simulink model "code"  (R2018b)
settings: Solver=VariableStepAuto  StartTime=0.0  StopTime=40.0  RelTol=1e-3
settings Model: Creator=Shubhi  LastModifiedBy=Shubhi

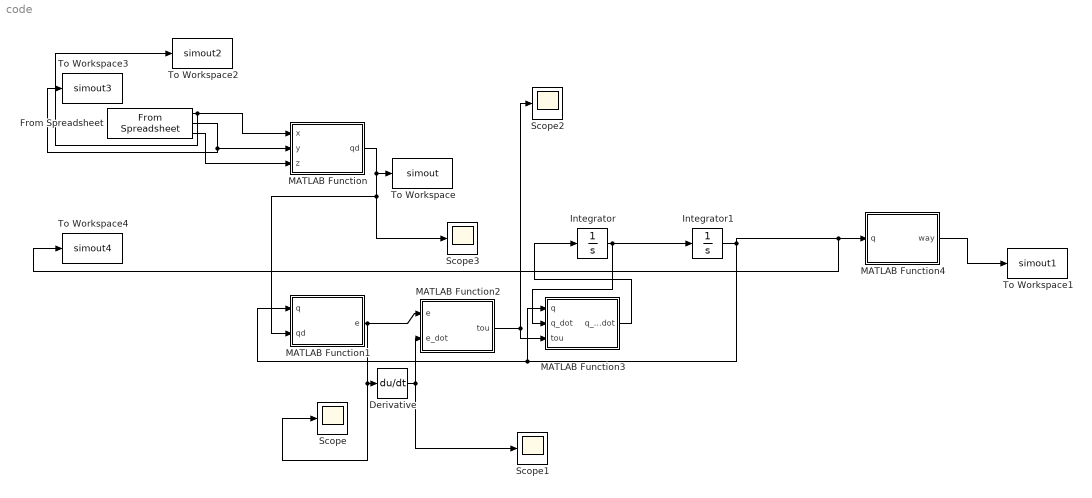
== system code ==
  Derivative : Derivative
  From Spreadsheet : FromSpreadsheet  FileName=C:\Users\Shubhi\Downloads\testdata.xlsx  SampleTime=0.5
  Integrator : Integrator  InitialCondition=[0;0;0;0]
  Integrator1 : Integrator  InitialCondition=[0;0;0;0]
  MATLAB Function : MATLAB Function  TreatAsAtomicUnit=on
  MATLAB Function1 : MATLAB Function  TreatAsAtomicUnit=on
  MATLAB Function2 : MATLAB Function  TreatAsAtomicUnit=on
  MATLAB Function3 : MATLAB Function  TreatAsAtomicUnit=on
  MATLAB Function4 : MATLAB Function  TreatAsAtomicUnit=on
  Scope{,1..3} (4 alike) : Scope
  To Workspace : ToWorkspace  VariableName=simout  SaveFormat=Timeseries  SampleTime=-1
  To Workspace1 : ToWorkspace  VariableName=simout1  SaveFormat=Timeseries  SampleTime=-1
  To Workspace2 : ToWorkspace  VariableName=simout2  SaveFormat=Timeseries  SampleTime=-1
  To Workspace3 : ToWorkspace  VariableName=simout3  SaveFormat=Timeseries  SampleTime=-1
  To Workspace4 : ToWorkspace  VariableName=simout4  SaveFormat=Timeseries  SampleTime=-1
  wires:
  From Spreadsheet/1 -> To Workspace2/1, MATLAB Function/1(x)
  From Spreadsheet/3 -> MATLAB Function/3(z)
  From Spreadsheet/2 -> To Workspace3/1, MATLAB Function/2(y)
  MATLAB Function/1(qd) -> Scope3/1, MATLAB Function1/2(qd), To Workspace/1
  MATLAB Function1/1(e) -> Scope/1, Derivative/1, MATLAB Function2/1(e)
  Derivative/1 -> Scope1/1, MATLAB Function2/2(e_dot)
  MATLAB Function2/1(tou) -> Scope2/1, MATLAB Function3/3(tou)
  Integrator/1 -> MATLAB Function3/2(q_dot), Integrator1/1
  MATLAB Function3/1(q_double_dot) -> Integrator/1
  Integrator1/1 -> To Workspace4/1, MATLAB Function4/1(q), MATLAB Function1/1(q), MATLAB Function3/1(q)
  MATLAB Function4/1(way) -> To Workspace1/1

== matlab function code/MATLAB Function1 ==
  data: q input; e output; qd input
function e=fcn(q, qd)
e=q-qd;

== matlab function code/MATLAB Function ==
  data: x input; qd output; y input; z input
function qd = fcn(x,y,z) 
l1=0.2;
l2=0.25;
theta1=acos(x/(x*x+y*y)^0.5) - acos((x^2+y^2+l1^2-l2^2)/(2*l1*(x^2+y^2)^(1/2))); 
theta2=acos(((x^2+y^2-l1^2-l2^2)/(2*l1*l2)));      
l0=0;

%a=y<0.2 | x<0;
%qd=[((-1)^(1+a)).*theta1;((-1)^(1+a)).*theta2;0;z-l0];
qd=[theta1;theta2;0;z-l0];

== matlab function code/MATLAB Function2 ==
  data: e input; tou output; e_dot input
function tou = fcn(e,e_dot)

 tou = -20*e-20*e_dot;

== matlab function code/MATLAB Function3 ==
  data: q_double_dot output; q input; q_dot input; tou input
function q_double_dot = fcn(q,q_dot,tou)

m1 = 20;
m2 = 15;
m3 = 15;
m4 = 0.5; 
 
l1 = 0.2;
l2 = 0.25; 
r1 = 0.1;
r2 = 0.125;

Iz1 = 0.27 ; 
 Iz2= 0.31;
Iz3 = 0.02;
Iz4 = 0.0001;
alpha =  Iz1+m1*r1^2+m2*l1^2+m3*l1^2+m4*l1^2;   
beta = Iz1+Iz2+Iz3+Iz4+l2^2*m3+l2^2*m4+r2^2*m2;
gamma=l1*l2*m3+l1*l2*m4+l1*m2*r2; 
delta = Iz3+Iz4;

g=9.8;
       
M=[alpha+beta+2*gamma*cos(q(2)), beta+gamma*cos(q(2)),delta,0;
    beta+gamma*cos(q(2)),beta, delta,0;
    delta,delta,delta,0;
    0,0,0,m4];

C=[-gamma*sin(q(2))*q_dot(2), -gamma*sin(q(2))*(q_dot(1)+q_dot(2)), 0, 0  ;
   -gamma*sin(q(2))*q_dot(1),0,0,0;
   0,0,0,0;
   0,0,0,0]; 

G=[0;0;0;m4*g];     
q_double_dot= (inv(M))* (tou-G-(C*q_dot));

== matlab function code/MATLAB Function4 ==
  data: q input; way output
function way = fcn(q)
   
x=0.2*cos(q(1))+0.25*cos(q(1)+q(2));
y=0.2*sin(q(1))+0.25*sin(q(1)+q(2));
              
z=q(4); 

way=[x,y,z]; 

plot3(x,y,z);
